simulink model "hazard_model"  (R2014a)
settings: Solver=ode45  StartTime=0.0  StopTime=5  RelTol=1e-3
libraries: simulink x1
settings Model: Creator=Divya M  LastModifiedBy=Divya M

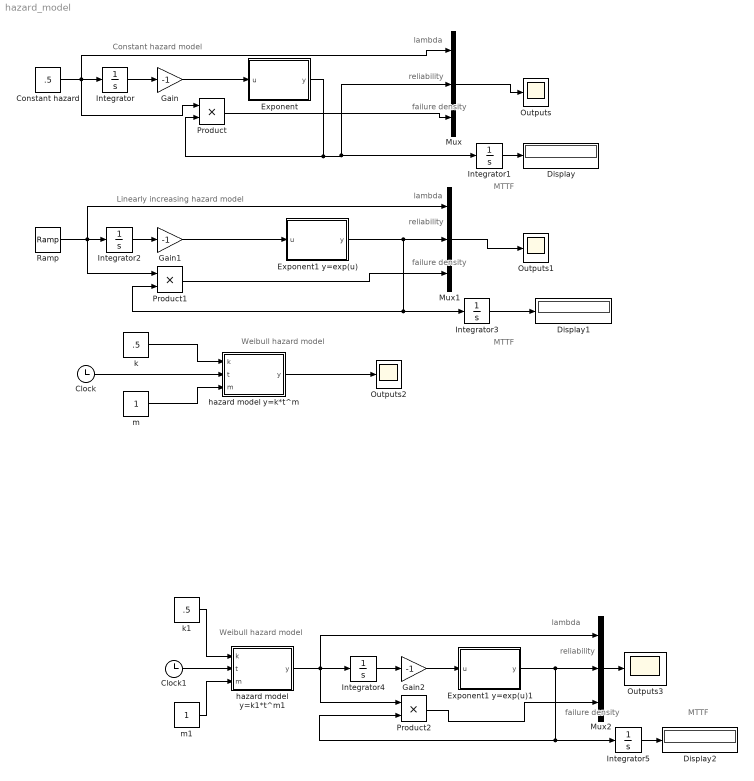
== system hazard_model ==
  note: Weibull hazard model
  note: Linearly increasing hazard model
  note: Constant hazard model
  note: MTTF
  note: failure
      | density
  note: reliability
  note: lambda
  note: MTTF
  note: failure
      | density
  note: reliability
  note: lambda
  note: Weibull hazard model
  note: MTTF
  note: failure
      | density
  note: reliability
  note: lambda
  Clock : Clock
  Clock1 : Clock
  Constant hazard : Constant  Value=.5
  Display : Display
  Display1 : Display
  Display2 : Display
  Exponent : MATLAB Function  TreatAsAtomicUnit=on
  Exponent1 y=exp(u) : MATLAB Function  TreatAsAtomicUnit=on
  Exponent1 y=exp(u)1 : MATLAB Function  TreatAsAtomicUnit=on
  Gain : Gain  Gain=-1
  Gain1 : Gain  Gain=-1
  Gain2 : Gain  Gain=-1
  Integrator{,1..5} (6 alike) : Integrator
  Mux : Mux  Inputs=3
  Mux1 : Mux  Inputs=3
  Mux2 : Mux  Inputs=3
  Outputs{,1..3} (4 alike) : Scope
      Outputs settings: YMin=0  YMax=1.1
      Outputs1 settings: YMin=0  YMax=1.12
      Outputs2 settings: YMin=0  YMax=2  SaveName=ScopeData2
      Outputs3 settings: YMin=0  YMax=1.12  SaveName=ScopeData3
  Product : Product
  Product1 : Product
  Product2 : Product
  Ramp : simulink/Sources/Ramp  slope=.5  start=0  X0=0
  hazard model y=k*t^m : MATLAB Function  TreatAsAtomicUnit=on
  hazard model y=k1*t^m1 : MATLAB Function  TreatAsAtomicUnit=on
  k : Constant  Value=.5
  k1 : Constant  Value=.5
  m : Constant
  m1 : Constant
  wires:
  Integrator/1 -> Gain/1
  Gain/1 -> Exponent/1(u)
  Exponent/1(y) -> Integrator1/1, Mux/2, Product/2
  Constant hazard/1 -> Product/1, Mux/1, Integrator/1
  Mux/1 -> Outputs/1
  Product/1 -> Mux/3
  Integrator2/1 -> Gain1/1
  Gain1/1 -> Exponent1 y=exp(u)/1(u)
  Exponent1 y=exp(u)/1(y) -> Mux1/2, Product1/2, Integrator3/1
  Ramp/1 -> Mux1/1, Product1/1, Integrator2/1
  Mux1/1 -> Outputs1/1
  Product1/1 -> Mux1/3
  Clock/1 -> hazard model y=k*t^m/2(t)
  k/1 -> hazard model y=k*t^m/1(k)
  m/1 -> hazard model y=k*t^m/3(m)
  hazard model y=k*t^m/1(y) -> Outputs2/1
  Integrator1/1 -> Display/1
  Integrator3/1 -> Display1/1
  Clock1/1 -> hazard model y=k1*t^m1/2(t)
  k1/1 -> hazard model y=k1*t^m1/1(k)
  m1/1 -> hazard model y=k1*t^m1/3(m)
  hazard model y=k1*t^m1/1(y) -> Product2/1, Mux2/1, Integrator4/1
  Integrator4/1 -> Gain2/1
  Gain2/1 -> Exponent1 y=exp(u)1/1(u)
  Exponent1 y=exp(u)1/1(y) -> Mux2/2, Product2/2, Integrator5/1
  Mux2/1 -> Outputs3/1
  Product2/1 -> Mux2/3
  Integrator5/1 -> Display2/1

== matlab function hazard_model/Exponent1 y=exp(u) ==
  data: u input; y output
function y = fcn(u)
%#codegen

y = exp(u);

== matlab function hazard_model/Exponent ==
  data: u input; y output
function y = fcn(u)
%#codegen

y = exp(u);

== matlab function hazard_model/hazard model y=k*t^m ==
  data: k input; y output; t input; m input
function y = fcn(k,t,m)
%#codegen

y = k*t^m;

== matlab function hazard_model/hazard model y=k1*t^m1 ==
  data: k input; y output; t input; m input
function y = fcn(k,t,m)
%#codegen

y = k*t^m;

== matlab function hazard_model/Exponent1 y=exp(u)1 ==
  data: u input; y output
function y = fcn(u)
%#codegen

y = exp(u);
